simulink model "mass_measurement_sim"  (R2025b)
settings: Solver=ode5  StartTime=0.0  StopTime=1.5  RelTol=1e-3
undefined symbols (not defined in the file or in its folder): National_Instruments, PCI, SampleTime
libraries: sldrtlib x6
settings Model: Creator=aie4-26  LastModifiedBy=David
settings HardwareCC: ProdBitPerLong=64.0  ProdHWDeviceType=Intel->x86-64 (Linux 64)
settings RTWCC: SystemTargetFile=sldrt.tlc  TemplateMakefile=sldrt.tmf  RTWCompilerOptimization=on  GPUComputeCapability=3.5  Description=Simulink Desktop Real-Time
settings CodeAppCC: MaxIdLength=95.0
settings SimulinkDesktopRealTimeCC: ExtModeTransport=0.0  ExtModeStaticAllocSize=1000000.0  TargetLibSuffix=_sldrt.a  TargetPreCompLibLocation=C:\Program Files\MATLAB\R2025b\toolbox\sldrt\lib\win64  MultiwordLength=2048.0  DynamicStringBufferSize=256.0  ParMdlRefBuildCompliant=on  PreserveMATLABNamespacesInGeneratedCode=on  SubcomponentCodeInterfacePackaging=Reusable function

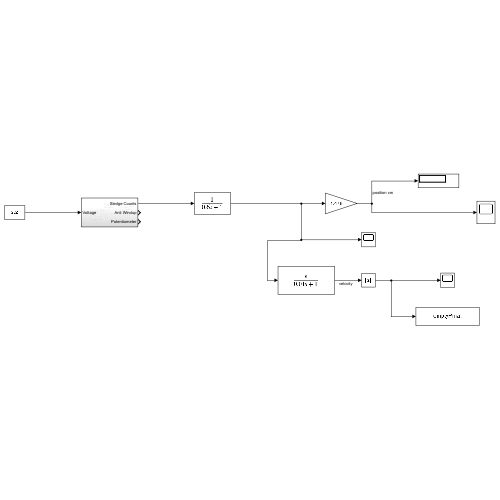
[thumbnail: Simulink's stored preview of the top-level diagram]
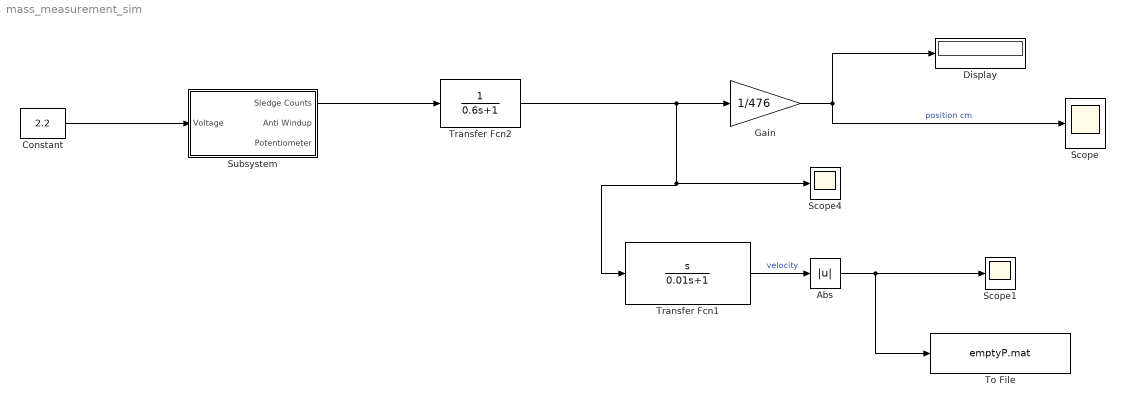
== system mass_measurement_sim ==
  Abs : Abs  SaturateOnIntegerOverflow=off
  Constant : Constant  Value=2.2
  Display : Display
  Gain : Gain  Gain=1/476
  Scope : Scope
      settings: ActiveDisplayYMinimum=-4.2733718487394947  ActiveDisplayYMaximum=38.460346638655459  DataLoggingVariableName=ScopeData4
  Scope1 : Scope
      settings: ActiveDisplayYMinimum=8630.4825544596952  ActiveDisplayYMaximum=8689.3155698777227  DataLoggingVariableName=ScopeData5
  Scope4 : Scope
      settings: ActiveDisplayYMinimum=-1387.084431678755  ActiveDisplayYMaximum=12483.759885108797  DataLoggingVariableName=ScopeData8
  Subsystem : Subsystem
  To File : ToFile  Filename=emptyP.mat  SaveFormat=Timeseries
  Transfer Fcn1 : TransferFcn  Numerator=[1 0]  Denominator=[0.01 1]
  Transfer Fcn2 : TransferFcn  Denominator=[0.6 1]
  wires:
  Gain/1 -> Display/1, Scope/1  "position cm"
  Transfer Fcn1/1 -> Abs/1  "velocity"
  Constant/1 -> Subsystem/1(Voltage)
  Abs/1 -> Scope1/1, To File/1
  Subsystem/1(Sledge Counts) -> Transfer Fcn2/1
  Transfer Fcn2/1 -> Transfer Fcn1/1, Scope4/1, Gain/1

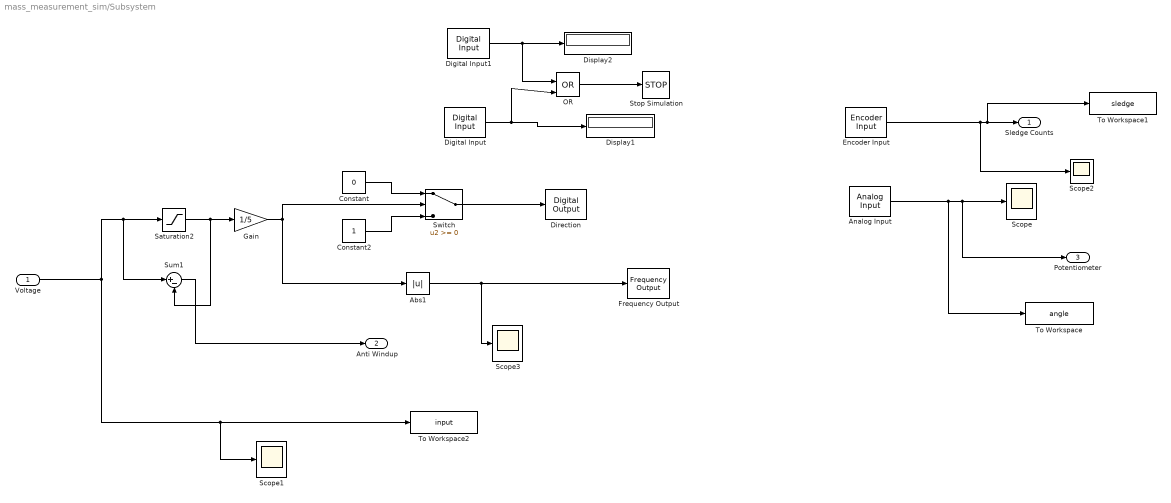
== system mass_measurement_sim/Subsystem ==
  Voltage : Inport
  Abs1 : Abs  SaturateOnIntegerOverflow=off
  Analog Input : sldrtlib/Analog Input  SampleTime=SampleTime  MaxMissedTicks=MaxMissedTicks  ShowMissedTicks=off  YieldWhenWaiting=off  DrvName=National_Instruments/PCI-6229  DrvAddress=4294967295  DrvOptions=[1 1 8192 2 3]  Channels=1  RangeMode=1  VoltRange=2  DataType=1
      settings: AttributesFormatString=National Instruments\nPCI-6229 [auto]
  Constant : Constant  Value=0  SampleTime=SampleTime
  Constant2 : Constant  SampleTime=SampleTime
  Digital Input : sldrtlib/Digital Input  SampleTime=0.1  MaxMissedTicks=10  ShowMissedTicks=off  YieldWhenWaiting=off  DrvName=National_Instruments/PCI-6229  DrvAddress=4294967295  DrvOptions=[1 1 8192 2 3]  Channels=2  BitMode=1  DataType=9
      settings: AttributesFormatString=National Instruments\nPCI-6229 [auto]
  Digital Input1 : sldrtlib/Digital Input  SampleTime=0.1  MaxMissedTicks=10  ShowMissedTicks=off  YieldWhenWaiting=off  DrvName=National_Instruments/PCI-6229  DrvAddress=4294967295  DrvOptions=[1 1 8192 2 3]  Channels=3  BitMode=1  DataType=9
      settings: AttributesFormatString=National Instruments\nPCI-6229 [auto]
  Direction : sldrtlib/Digital Output  SampleTime=SampleTime  MaxMissedTicks=MaxMissedTicks  ShowMissedTicks=off  YieldWhenWaiting=off  DrvName=National_Instruments/PCI-6229  DrvAddress=4294967295  DrvOptions=[1 1 8192 2 3]  Channels=1  BitMode=1  InitialValue=0  FinalValue=0
      settings: AttributesFormatString=National Instruments\nPCI-6229 [auto]
  Display1 : Display
  Display2 : Display
  Encoder Input : sldrtlib/Encoder Input  SampleTime=0.001  MaxMissedTicks=10000000  ShowMissedTicks=off  YieldWhenWaiting=off  DrvName=National_Instruments/PCI-6229  DrvAddress=4294967295  DrvOptions=[1 1 8192 2 3]  Channels=1  QuadMode=2  IndexPulse=2  InputFilter=Inf  DataType=1
      settings: AttributesFormatString=National Instruments\nPCI-6229 [auto]
  Frequency Output : sldrtlib/Frequency Output  SampleTime=SampleTime  MaxMissedTicks=MaxMissedTicks  ShowMissedTicks=off  YieldWhenWaiting=off  DrvName=National_Instruments/PCI-6229  DrvAddress=4294967295  DrvOptions=[1 1 8192 2 3]  Channels=2  FrequencySource=1  Frequency=10000  FrequencyFinalValue=[]  DutySource=2  Duty=0  DutyFinalValue=0
      settings: AttributesFormatString=National Instruments\nPCI-6229 [auto]
  Gain : Gain  Gain=1/5
  OR : Logic  Operator=OR  IconShape=distinctive  AllPortsSameDT=off  OutDataTypeStr=boolean
  Saturation2 : Saturate  UpperLimit=2.5  LowerLimit=-2.5
  Scope{,1..3} (4 alike) : Scope
      Scope settings: ActiveDisplayYMinimum=-1.7267364976437558  ActiveDisplayYMaximum=6.2920540572750241
      Scope1 settings: ActiveDisplayYMinimum=-3.75  ActiveDisplayYMaximum=3.75  DataLoggingVariableName=ScopeData2
      Scope2 settings: ActiveDisplayYMinimum=-935.75  ActiveDisplayYMaximum=8421.75  DataLoggingVariableName=ScopeData3
      Scope3 settings: ActiveDisplayYMinimum=-0.0625  ActiveDisplayYMaximum=0.5625
  Stop Simulation : Stop
  Sum1 : Sum  Inputs=|+-
  Switch : Switch  SaturateOnIntegerOverflow=off  InputSameDT=off
  To Workspace : ToWorkspace  VariableName=angle  SaveFormat=Timeseries  SampleTime=-1
  To Workspace1 : ToWorkspace  VariableName=sledge  SaveFormat=Timeseries  SampleTime=-1
  To Workspace2 : ToWorkspace  VariableName=input  SaveFormat=Timeseries  SampleTime=-1
  Sledge Counts : Outport
  Anti Windup : Outport  Port=2
  Potentiometer : Outport  Port=3
  wires:
  Digital Input/1 -> OR/2, Display1/1
  Abs1/1 -> Scope3/1, Frequency Output/1
  Constant/1 -> Switch/1
  Digital Input1/1 -> OR/1, Display2/1
  Voltage/1 -> Scope1/1, To Workspace2/1, Sum1/1, Saturation2/1
  Analog Input/1 -> To Workspace/1, Potentiometer/1, Scope/1
  OR/1 -> Stop Simulation/1
  Saturation2/1 -> Sum1/2, Gain/1
  Constant2/1 -> Switch/3
  Sum1/1 -> Anti Windup/1
  Encoder Input/1 -> Scope2/1, Sledge Counts/1, To Workspace1/1
  Switch/1 -> Direction/1
  Gain/1 -> Abs1/1, Switch/2
